simulink subsystem "DCServoMotor_SubSystem"  (R2020b)
settings: Solver=VariableStepAuto  StartTime=0.0  StopTime=10.0  RelTol=1e-3
undefined symbols (not defined in the file or in its folder): sens
settings Model: Creator=umberto  LastModifiedBy=umbe

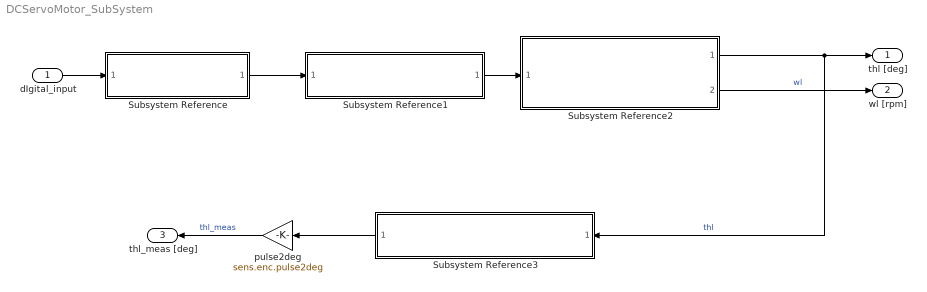
== system DCServoMotor_SubSystem ==
  dIgital_input : Inport
  Subsystem Reference : Subsystem  ReferencedSubsystem=DAC_SubSystem
  Subsystem Reference1 : Subsystem  ReferencedSubsystem=Driver_SubSystem
  Subsystem Reference2 : Subsystem  ReferencedSubsystem=DCGearbox_SubSystem
  Subsystem Reference3 : Subsystem  ReferencedSubsystem=Encoder_SubSystem
  pulse2deg : Gain  Gain=sens.enc.pulse2deg
  thl [deg] : Outport
  wl [rpm] : Outport  Port=2
  thl_meas [deg] : Outport  Port=3
  wires:
  dIgital_input/1 -> Subsystem Reference/1
  Subsystem Reference1/1 -> Subsystem Reference2/1
  Subsystem Reference2/1 -> thl [deg]/1, Subsystem Reference3/1  "thl"
  Subsystem Reference2/2 -> wl [rpm]/1  "wl"
  Subsystem Reference3/1 -> pulse2deg/1
  pulse2deg/1 -> thl_meas [deg]/1  "thl_meas"
  Subsystem Reference/1 -> Subsystem Reference1/1
